simulink model "backstep"  (R2023a)
settings: Solver=VariableStepAuto  StartTime=0.0  StopTime=50  RelTol=1e-3
libraries: simulink x2
settings Model: Creator=30296  LastModifiedBy=30296

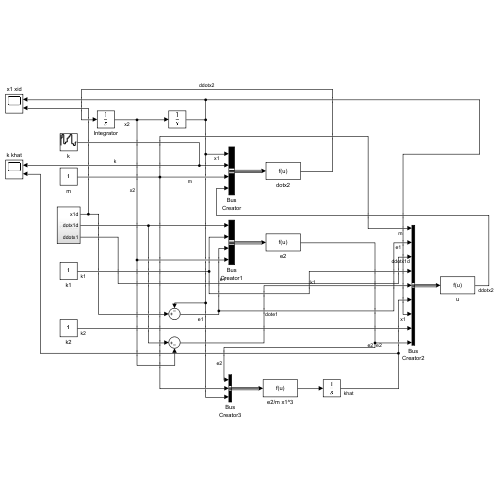
[thumbnail: Simulink's stored preview of the top-level diagram]
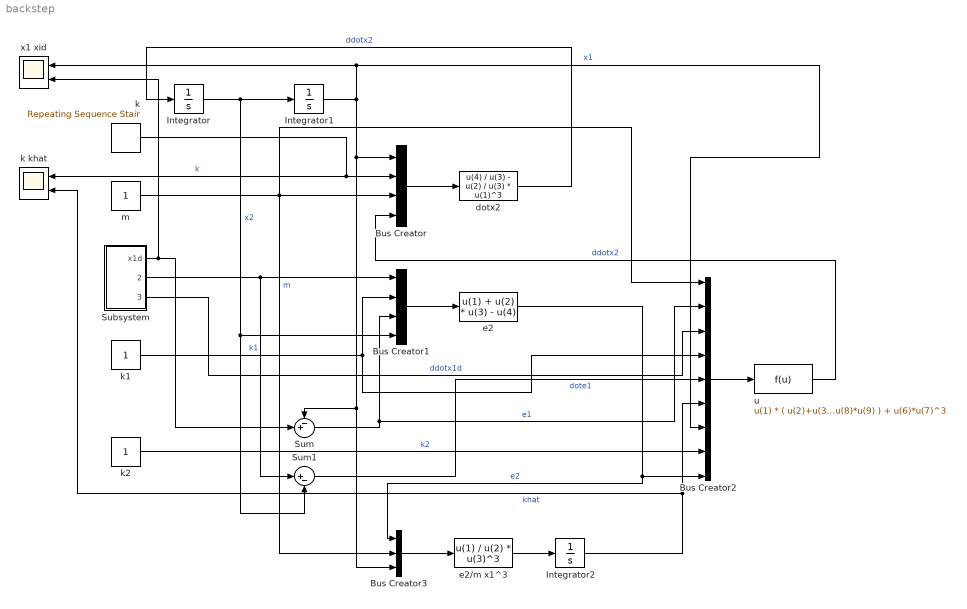
== system backstep ==
  Bus Creator : BusCreator  Inputs=4
  Bus Creator1 : BusCreator  Inputs=4
  Bus Creator2 : BusCreator  Inputs=9
  Bus Creator3 : BusCreator  Inputs=3
  Integrator : Integrator
  Integrator1 : Integrator
  Integrator2 : Integrator
  Subsystem : Subsystem
  Sum : Sum  Inputs=-+|
  Sum1 : Sum  Inputs=|+-
  dotx2 : Fcn  Expr=u(4) / u(3) - u(2) / u(3) * u(1)^3
  e2 : Fcn  Expr=u(1) + u(2) * u(3) - u(4)
  e2/m x1^3 : Fcn  Expr=u(1) / u(2) * u(3)^3
  k : simulink/Sources/Repeating Sequence Stair  OutValues=[8 10 5 6 8 9 10 5 4 6].'  tsamp=5  OutMin=[]  OutMax=[]  OutDataTypeStr=double  OutputDataTypeScalingMode=double  OutDataType=fixdt(0,8)  ConRadixGroup=Best Precision: Vector-wise  OutScaling=2^-12
  k khat : Scope  NumInputPorts=2
  k1 : Constant
  k2 : Constant
  m : Constant
  u : Fcn  Expr=u(1) * ( u(2)+u(3)+u(4)*u(5)+u(8)*u(9) ) + u(6)*u(7)^3
  x1 xid : Scope  NumInputPorts=2
  wires:
  Integrator/1 -> Integrator1/1, Sum1/2, Bus Creator1/4  "x2"
  Integrator1/1 -> x1 xid/1, Bus Creator2/7, Sum/1, Bus Creator3/3, Bus Creator/1  "x1"
  dotx2/1 -> Integrator/1  "ddotx2"
  k/1 -> k khat/1, Bus Creator/2  "k"
  m/1 -> Bus Creator2/1, Bus Creator/3, Bus Creator3/2  "m"
  Bus Creator/1 -> dotx2/1
  Subsystem/1(x1d) -> Sum/2, x1 xid/2
  Subsystem/2(dotx1d) -> Sum1/1, Bus Creator1/1
  k1/1 -> Bus Creator2/4, Bus Creator1/2  "k1"
  Sum/1 -> Bus Creator2/2, Bus Creator1/3  "e1"
  Bus Creator1/1 -> e2/1
  Bus Creator2/1 -> u/1
  Subsystem/3(ddotx1) -> Bus Creator2/3  "ddotx1d"
  Sum1/1 -> Bus Creator2/5  "dote1"
  e2/1 -> Bus Creator3/1, Bus Creator2/9  "e2"
  e2/m x1^3/1 -> Integrator2/1
  Integrator2/1 -> k khat/2, Bus Creator2/6  "khat"
  Bus Creator3/1 -> e2/m x1^3/1
  k2/1 -> Bus Creator2/8  "k2"
  u/1 -> Bus Creator/4  "ddotx2"

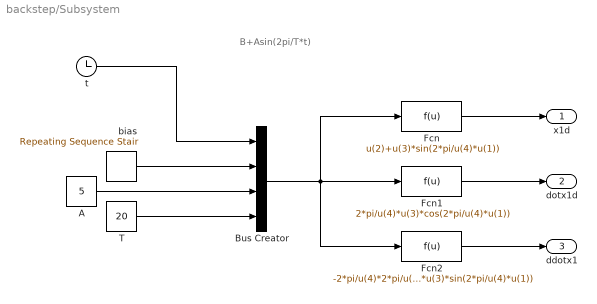
== system backstep/Subsystem ==
  note: B+Asin(2pi/T*t)
  A : Constant  Value=5
  Bus Creator : BusCreator  Inputs=4
  Fcn : Fcn  Expr=u(2)+u(3)*sin(2*pi/u(4)*u(1))
  Fcn1 : Fcn  Expr=2*pi/u(4)*u(3)*cos(2*pi/u(4)*u(1))
  Fcn2 : Fcn  Expr=-2*pi/u(4)*2*pi/u(4)*u(3)*sin(2*pi/u(4)*u(1))
  T : Constant  Value=20
  bias : simulink/Sources/Repeating Sequence Stair  OutValues=[0 1 2 3 4].'  tsamp=10  OutMin=[]  OutMax=[]  OutDataTypeStr=double  OutputDataTypeScalingMode=double  OutDataType=fixdt(0,8)  ConRadixGroup=Best Precision: Vector-wise  OutScaling=2^-12
  t : Clock
  x1d : Outport
  dotx1d : Outport  Port=2
  ddotx1 : Outport  Port=3
  wires:
  Fcn/1 -> x1d/1
  Fcn1/1 -> dotx1d/1
  Fcn2/1 -> ddotx1/1
  Bus Creator/1 -> Fcn1/1, Fcn2/1, Fcn/1
  t/1 -> Bus Creator/1
  bias/1 -> Bus Creator/2
  A/1 -> Bus Creator/3
  T/1 -> Bus Creator/4
